simulink model "diff_flatness_linear_nl"  (R2022b)
settings: Solver=FixedStepAuto  StartTime=0.0  StopTime=15  RelTol=1e-3
model workspace (MAT data in the model file):
  kp = Simulink.Parameter
  kp.DataType = 'auto'
  kp.Complexity = 'real'
  kp.Dimensions = [0 0]
libraries: robotmobilelib x5, dspsigops x5
settings Model: Creator=RichiRettore  LastModifiedBy=RichiRettore
settings OptimizationCC: ReuseModelBlockBuffer=on

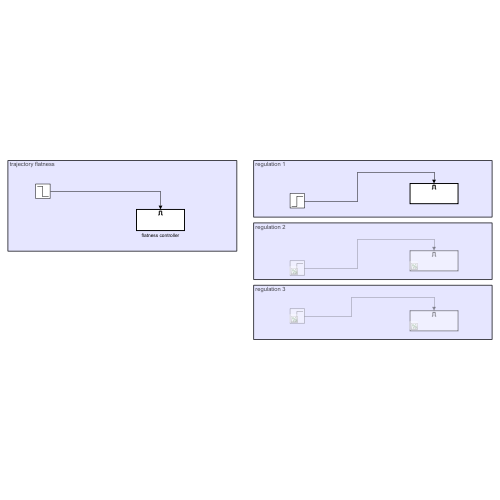
[thumbnail: Simulink's stored preview of the top-level diagram]
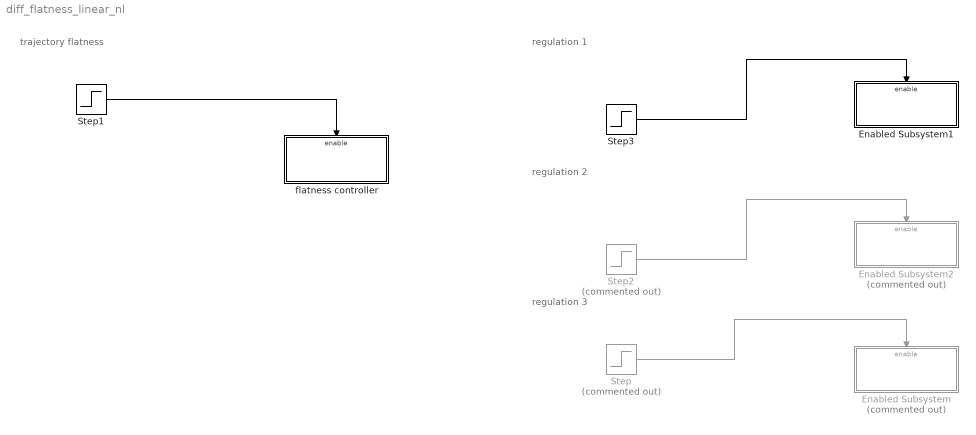
== system diff_flatness_linear_nl ==
  note: regulation 3
  note: regulation 2
  note: regulation 1
  note: trajectory flatness
  Enabled Subsystem : Subsystem  Commented=on  TreatAsAtomicUnit=on
  Enabled Subsystem1 : Subsystem  TreatAsAtomicUnit=on
  Enabled Subsystem2 : Subsystem  Commented=on  TreatAsAtomicUnit=on
  Step : Step  Commented=on  Time=10  SampleTime=0
  Step1 : Step  Time=10  Before=1  After=0  SampleTime=0
  Step2 : Step  Commented=on  Time=10  SampleTime=0
  Step3 : Step  Time=10  SampleTime=0
  flatness controller : Subsystem  TreatAsAtomicUnit=on
  wires:
  Step2/1 -> Enabled Subsystem2/Enable
  Step1/1 -> flatness controller/Enable
  Step/1 -> Enabled Subsystem/Enable
  Step3/1 -> Enabled Subsystem1/Enable

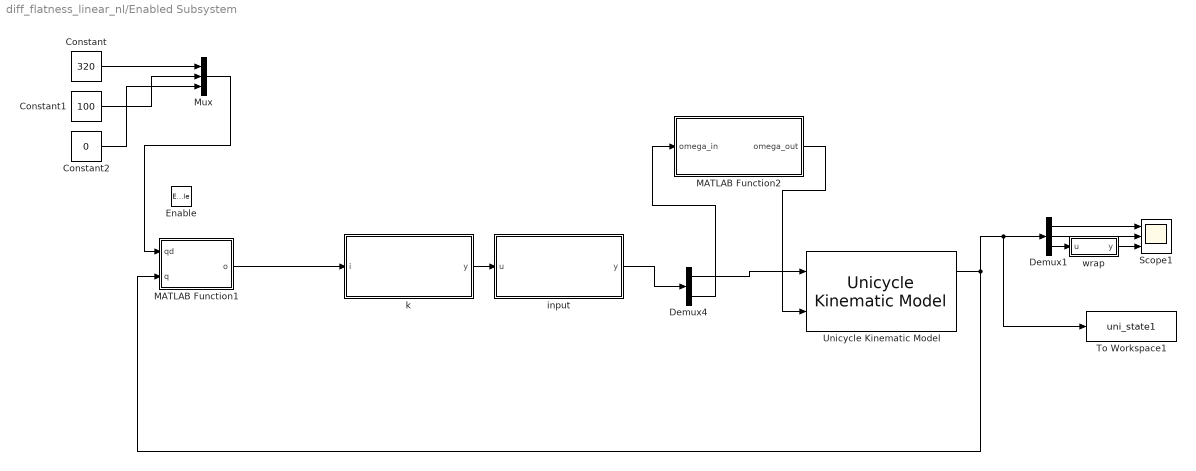
== system diff_flatness_linear_nl/Enabled Subsystem ==
  Enable : EnablePort
  Constant : Constant  Value=320
  Constant1 : Constant  Value=100
  Constant2 : Constant  Value=0
  Demux1 : Demux  Outputs=3
  Demux4 : Demux  Outputs=2
  MATLAB Function1 : MATLAB Function  TreatAsAtomicUnit=on
  MATLAB Function2 : MATLAB Function  TreatAsAtomicUnit=on
  Mux : Mux  Inputs=3
  Scope1 : Scope  NumInputPorts=3
  To Workspace1 : ToWorkspace  VariableName=uni_state1  SaveFormat=Structure With Time  SampleTime=0.001
  Unicycle Kinematic Model : robotmobilelib/Unicycle Kinematic Model  VehicleInputs=Vehicle Speed & Heading Angular Velocity  WheelRadius=2  WheelSpeedRange=[-Inf Inf]  InitialState=[125,60,0]  SimulateUsing=Interpreted execution
  input : MATLAB Function  TreatAsAtomicUnit=on
  k : MATLAB Function  TreatAsAtomicUnit=on
  wrap : MATLAB Function  TreatAsAtomicUnit=on
  wires:
  Constant/1 -> Mux/1
  Constant1/1 -> Mux/2
  Constant2/1 -> Mux/3
  Demux1/2 -> Scope1/2
  wrap/1(y) -> Scope1/3
  Unicycle Kinematic Model/1 -> To Workspace1/1, Demux1/1, MATLAB Function1/2(q)
  input/1(y) -> Demux4/1
  Demux1/3 -> wrap/1(u)
  k/1(y) -> input/1(u)
  Demux1/1 -> Scope1/1
  MATLAB Function1/1(o) -> k/1(i)
  Demux4/1 -> Unicycle Kinematic Model/1
  Mux/1 -> MATLAB Function1/1(qd)
  Demux4/2 -> MATLAB Function2/1(omega_in)
  MATLAB Function2/1(omega_out) -> Unicycle Kinematic Model/2

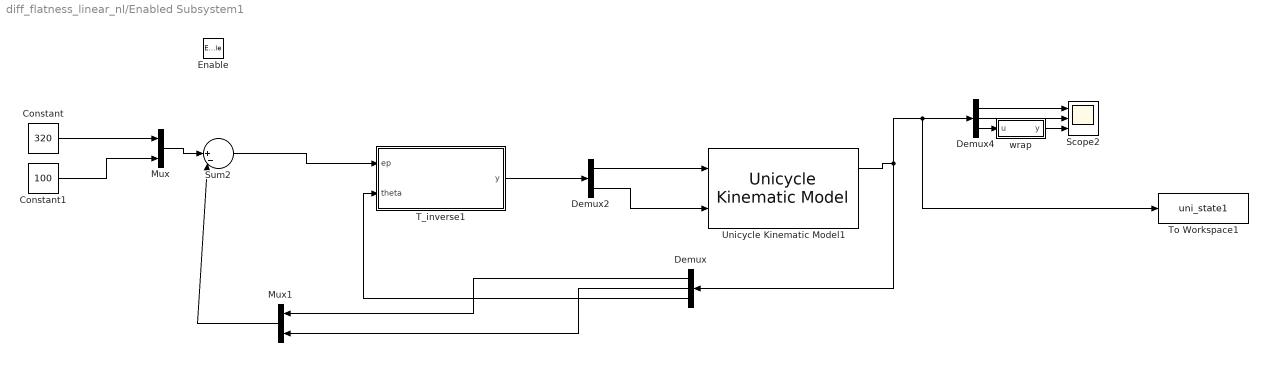
== system diff_flatness_linear_nl/Enabled Subsystem1 ==
  Enable : EnablePort
  Constant : Constant  Value=320
  Constant1 : Constant  Value=100
  Demux : Demux  Outputs=3
  Demux2 : Demux  Outputs=2
  Demux4 : Demux  Outputs=3
  Mux : Mux  Inputs=2
  Mux1 : Mux  Inputs=2
  Scope2 : Scope  NumInputPorts=3
  Sum2 : Sum  Inputs=||+-|
  T_inverse1 : MATLAB Function  TreatAsAtomicUnit=on
  To Workspace1 : ToWorkspace  VariableName=uni_state1  SaveFormat=Structure With Time  SampleTime=0.001
  Unicycle Kinematic Model1 : robotmobilelib/Unicycle Kinematic Model  VehicleInputs=Vehicle Speed & Heading Angular Velocity  WheelRadius=2  WheelSpeedRange=[-Inf Inf]  InitialState=[125,60,0]  SimulateUsing=Interpreted execution
  wrap : MATLAB Function  TreatAsAtomicUnit=on
  wires:
  wrap/1(y) -> Scope2/3
  Demux4/1 -> Scope2/1
  Demux4/2 -> Scope2/2
  Demux4/3 -> wrap/1(u)
  Sum2/1 -> T_inverse1/1(ep)
  Demux/1 -> Mux1/1
  Demux2/2 -> Unicycle Kinematic Model1/2
  Mux1/1 -> Sum2/2
  Demux2/1 -> Unicycle Kinematic Model1/1
  Unicycle Kinematic Model1/1 -> To Workspace1/1, Demux4/1, Demux/1
  T_inverse1/1(y) -> Demux2/1
  Demux/2 -> Mux1/2
  Demux/3 -> T_inverse1/2(theta)
  Constant1/1 -> Mux/2
  Constant/1 -> Mux/1
  Mux/1 -> Sum2/1

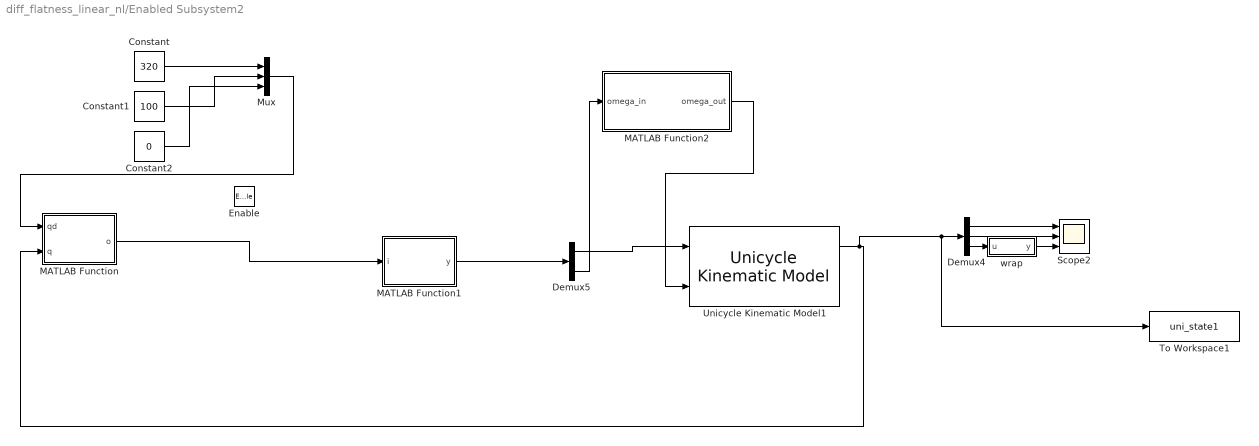
== system diff_flatness_linear_nl/Enabled Subsystem2 ==
  Enable : EnablePort
  Constant : Constant  Value=320
  Constant1 : Constant  Value=100
  Constant2 : Constant  Value=0
  Demux4 : Demux  Outputs=3
  Demux5 : Demux  Outputs=2
  MATLAB Function : MATLAB Function  TreatAsAtomicUnit=on
  MATLAB Function1 : MATLAB Function  TreatAsAtomicUnit=on
  MATLAB Function2 : MATLAB Function  TreatAsAtomicUnit=on
  Mux : Mux  Inputs=3
  Scope2 : Scope  NumInputPorts=3
  To Workspace1 : ToWorkspace  VariableName=uni_state1  SaveFormat=Structure With Time  SampleTime=0.001
  Unicycle Kinematic Model1 : robotmobilelib/Unicycle Kinematic Model  VehicleInputs=Vehicle Speed & Heading Angular Velocity  WheelRadius=2  WheelSpeedRange=[-Inf Inf]  InitialState=[125,60,0]  SimulateUsing=Interpreted execution
  wrap : MATLAB Function  TreatAsAtomicUnit=on
  wires:
  Demux5/1 -> Unicycle Kinematic Model1/1
  wrap/1(y) -> Scope2/3
  MATLAB Function/1(o) -> MATLAB Function1/1(i)
  MATLAB Function1/1(y) -> Demux5/1
  Demux4/1 -> Scope2/1
  Demux4/2 -> Scope2/2
  Demux4/3 -> wrap/1(u)
  Unicycle Kinematic Model1/1 -> To Workspace1/1, Demux4/1, MATLAB Function/2(q)
  Constant/1 -> Mux/1
  Constant1/1 -> Mux/2
  Constant2/1 -> Mux/3
  Mux/1 -> MATLAB Function/1(qd)
  Demux5/2 -> MATLAB Function2/1(omega_in)
  MATLAB Function2/1(omega_out) -> Unicycle Kinematic Model1/2

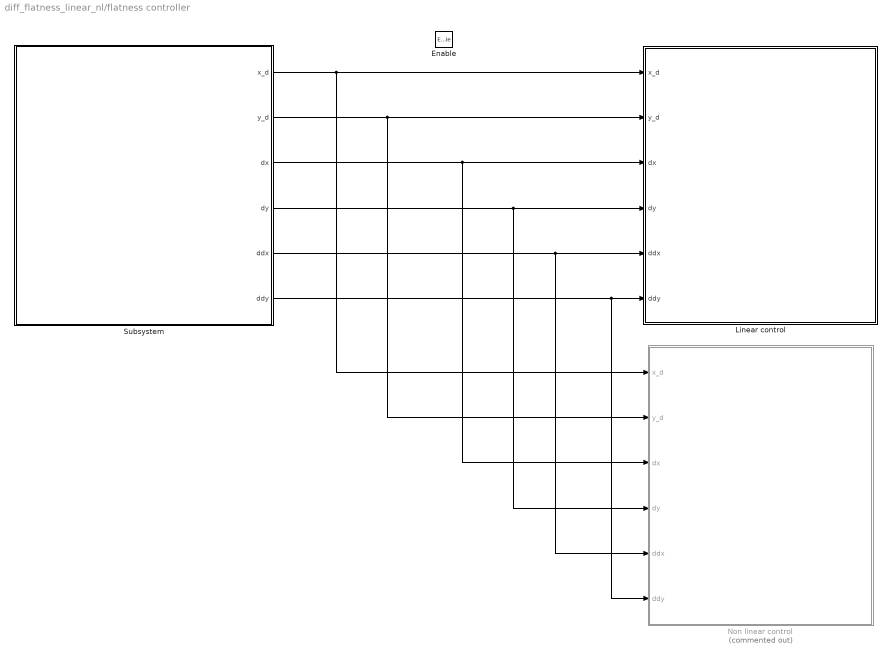
== system diff_flatness_linear_nl/flatness controller ==
  Enable : EnablePort
  Linear control : Subsystem
  Non linear control : Subsystem  Commented=on
  Subsystem : Subsystem
  wires:
  Subsystem/1(x_d) -> Non linear control/1(x_d), Linear control/1(x_d)
  Subsystem/2(y_d) -> Non linear control/2(y_d), Linear control/2(y_d)
  Subsystem/3(dx) -> Non linear control/3(dx), Linear control/3(dx)
  Subsystem/4(dy) -> Non linear control/4(dy), Linear control/4(dy)
  Subsystem/5(ddx) -> Non linear control/5(ddx), Linear control/5(ddx)
  Subsystem/6(ddy) -> Non linear control/6(ddy), Linear control/6(ddy)

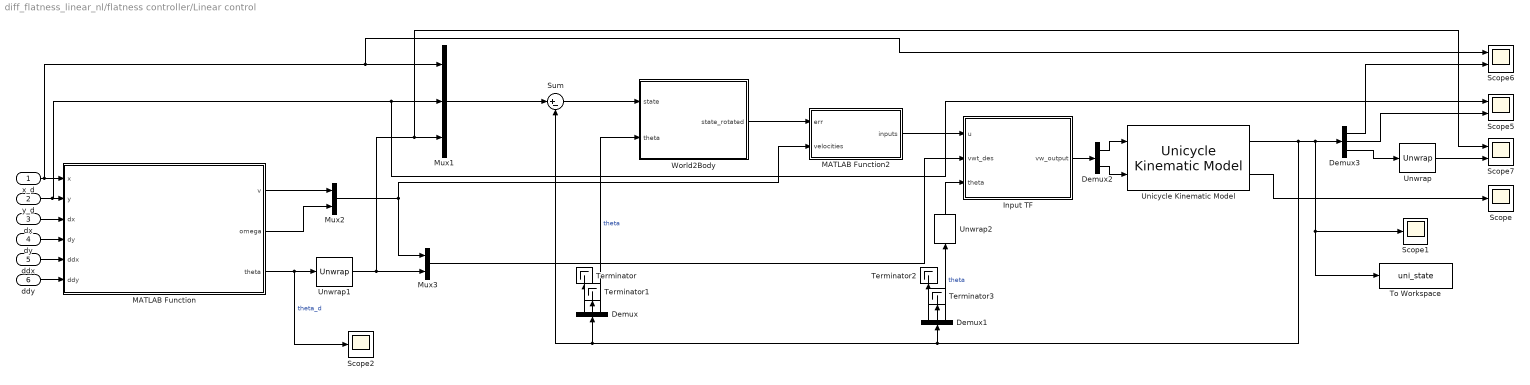
== system diff_flatness_linear_nl/flatness controller/Linear control ==
  x_d : Inport
  y_d : Inport  Port=2
  dx : Inport  Port=3
  dy : Inport  Port=4
  ddx : Inport  Port=5
  ddy : Inport  Port=6
  Demux : Demux  Outputs=3
  Demux1 : Demux  Outputs=3
  Demux2 : Demux  Outputs=2
  Demux3 : Demux  Outputs=3
  Input TF : MATLAB Function  TreatAsAtomicUnit=on
  MATLAB Function : MATLAB Function  TreatAsAtomicUnit=on
  MATLAB Function2 : MATLAB Function  TreatAsAtomicUnit=on
  Mux1 : Mux  Inputs=3
  Mux2 : Mux  Inputs=2
  Mux3 : Mux  Inputs=2
  Scope : Scope
  Scope1 : Scope
  Scope2 : Scope
  Scope5 : Scope  NumInputPorts=2
  Scope6 : Scope  NumInputPorts=2
  Scope7 : Scope  NumInputPorts=2
  Sum : Sum  Inputs=|+-
  Terminator{,1..3} (4 alike) : Terminator
  To Workspace : ToWorkspace  VariableName=uni_state  SaveFormat=Structure With Time  SampleTime=0.01
  Unicycle Kinematic Model : robotmobilelib/Unicycle Kinematic Model  VehicleInputs=Vehicle Speed & Heading Angular Velocity  WheelRadius=0.1  WheelSpeedRange=[-Inf Inf]  InitialState=[125; 60; 0]  SimulateUsing=Interpreted execution
  Unwrap : dspsigops/Unwrap  tol=pi  running=off
  Unwrap1 : dspsigops/Unwrap  tol=pi  running=off
  Unwrap2 : dspsigops/Unwrap  tol=pi  running=off
  World2Body : MATLAB Function  TreatAsAtomicUnit=on
  wires:
  Unicycle Kinematic Model/1 -> To Workspace/1, Scope1/1, Demux3/1, Sum/2, Demux/1, Demux1/1
  MATLAB Function/2(omega) -> Mux2/2
  dx/1 -> MATLAB Function/3(dx)
  Demux/3 -> World2Body/2(theta)  "theta"
  x_d/1 -> Scope6/1, Mux1/1, MATLAB Function/1(x)
  ddx/1 -> MATLAB Function/5(ddx)
  Sum/1 -> World2Body/1(state)
  World2Body/1(state_rotated) -> MATLAB Function2/1(err)
  Demux2/1 -> Unicycle Kinematic Model/1
  MATLAB Function2/1(inputs) -> Input TF/1(u)
  Demux2/2 -> Unicycle Kinematic Model/2
  Input TF/1(vw_output) -> Demux2/1
  Mux1/1 -> Sum/1
  MATLAB Function/3(theta) -> Unwrap1/1, Scope2/1  "theta_d"
  y_d/1 -> Scope5/1, Mux1/2, MATLAB Function/2(y)
  Demux3/1 -> Scope6/2
  Mux2/1 -> MATLAB Function2/2(velocities), Mux3/1
  Mux3/1 -> Input TF/2(vwt_des)
  Demux3/2 -> Scope5/2
  Unicycle Kinematic Model/2 -> Scope/1
  MATLAB Function/1(v) -> Mux2/1
  ddy/1 -> MATLAB Function/6(ddy)
  dy/1 -> MATLAB Function/4(dy)
  Demux/1 -> Terminator/1
  Demux/2 -> Terminator1/1
  Demux1/1 -> Terminator2/1
  Demux1/2 -> Terminator3/1
  Demux3/3 -> Unwrap/1
  Unwrap/1 -> Scope7/2
  Unwrap1/1 -> Scope7/1, Mux1/3, Mux3/2
  Demux1/3 -> Unwrap2/1  "theta"
  Unwrap2/1 -> Input TF/3(theta)

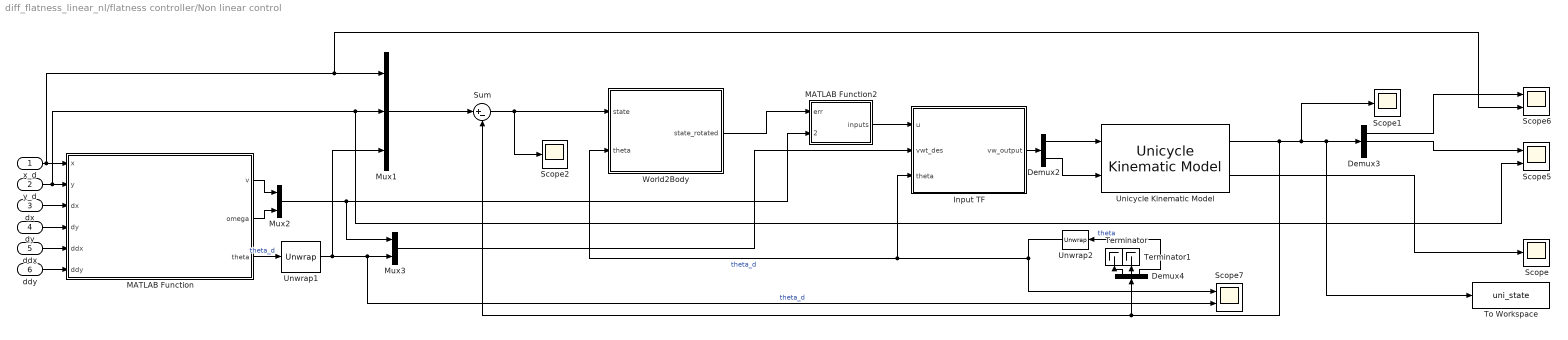
== system diff_flatness_linear_nl/flatness controller/Non linear control ==
  x_d : Inport
  y_d : Inport  Port=2
  dx : Inport  Port=3
  dy : Inport  Port=4
  ddx : Inport  Port=5
  ddy : Inport  Port=6
  Demux2 : Demux  Outputs=2
  Demux3 : Demux  Outputs=3
  Demux4 : Demux  Outputs=3
  Input TF : MATLAB Function  TreatAsAtomicUnit=on
  MATLAB Function : MATLAB Function  TreatAsAtomicUnit=on
  MATLAB Function2 : MATLAB Function  TreatAsAtomicUnit=on
  Mux1 : Mux  Inputs=3
  Mux2 : Mux  Inputs=2
  Mux3 : Mux  Inputs=2
  Scope : Scope
  Scope1 : Scope
  Scope2 : Scope
  Scope5 : Scope  NumInputPorts=2
  Scope6 : Scope  NumInputPorts=2
  Scope7 : Scope  NumInputPorts=2
  Sum : Sum  Inputs=|+-
  Terminator : Terminator
  Terminator1 : Terminator
  To Workspace : ToWorkspace  VariableName=uni_state  SaveFormat=Structure With Time  SampleTime=0.1
  Unicycle Kinematic Model : robotmobilelib/Unicycle Kinematic Model  VehicleInputs=Vehicle Speed & Heading Angular Velocity  WheelRadius=0.1  WheelSpeedRange=[-Inf Inf]  InitialState=[125; 60; 0]  SimulateUsing=Interpreted execution
  Unwrap1 : dspsigops/Unwrap  tol=pi  InputProcessing=Columns as channels (frame based)  running=off
  Unwrap2 : dspsigops/Unwrap  tol=pi  InputProcessing=Columns as channels (frame based)  running=off
  World2Body : MATLAB Function  TreatAsAtomicUnit=on
  wires:
  MATLAB Function/2(omega) -> Mux2/2
  dx/1 -> MATLAB Function/3(dx)
  x_d/1 -> Scope6/2, Mux1/1, MATLAB Function/1(x)
  ddx/1 -> MATLAB Function/5(ddx)
  Sum/1 -> World2Body/1(state), Scope2/1
  World2Body/1(state_rotated) -> MATLAB Function2/1(err)
  Demux2/1 -> Unicycle Kinematic Model/1
  MATLAB Function2/1(inputs) -> Input TF/1(u)
  Demux2/2 -> Unicycle Kinematic Model/2
  Input TF/1(vw_output) -> Demux2/1
  Mux1/1 -> Sum/1
  y_d/1 -> Scope5/2, Mux1/2, MATLAB Function/2(y)
  Demux3/1 -> Scope6/1
  Mux2/1 -> Mux3/1, MATLAB Function2/2(velocities)
  Mux3/1 -> Input TF/2(vwt_des)
  Demux3/2 -> Scope5/1
  Unicycle Kinematic Model/2 -> Scope/1
  MATLAB Function/1(v) -> Mux2/1
  ddy/1 -> MATLAB Function/6(ddy)
  dy/1 -> MATLAB Function/4(dy)
  MATLAB Function/3(theta) -> Unwrap1/1  "theta_d"
  Demux4/3 -> Unwrap2/1  "theta"
  Unwrap1/1 -> Mux1/3, Mux3/2, Scope7/2  "theta_d"
  Unicycle Kinematic Model/1 -> Demux4/1, Sum/2, To Workspace/1, Demux3/1, Scope1/1
  Unwrap2/1 -> Scope7/1, Input TF/3(theta), World2Body/2(theta)  "theta_d"
  Demux4/1 -> Terminator/1
  Demux4/2 -> Terminator1/1

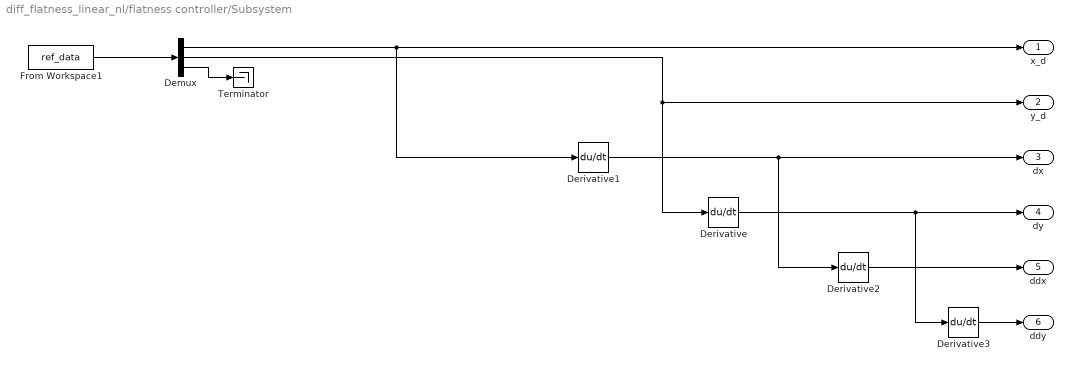
== system diff_flatness_linear_nl/flatness controller/Subsystem ==
  Demux : Demux  Outputs=3
  Derivative{,1..3} (4 alike) : Derivative
  From Workspace1 : FromWorkspace  VariableName=ref_data
  Terminator : Terminator
  x_d : Outport
  y_d : Outport  Port=2
  dx : Outport  Port=3
  dy : Outport  Port=4
  ddx : Outport  Port=5
  ddy : Outport  Port=6
  wires:
  Demux/3 -> Terminator/1
  Derivative/1 -> dy/1, Derivative3/1
  Derivative3/1 -> ddy/1
  Derivative1/1 -> dx/1, Derivative2/1
  From Workspace1/1 -> Demux/1
  Demux/1 -> x_d/1, Derivative1/1
  Demux/2 -> y_d/1, Derivative/1
  Derivative2/1 -> ddx/1

== matlab function diff_flatness_linear_nl/Enabled Subsystem/MATLAB Function2 ==
  data: omega_in input; omega_out output
function omega_out = check_omega(omega_in)
    % Check if omega (angular velocity) is finite
    if ~isfinite(omega_in)
        omega_out = 0;  % Set omega to a default value, e.g., 0 if it is NaN or Inf
    else
        omega_out = omega_in;  % Otherwise, pass the input value
    end
end

== matlab function diff_flatness_linear_nl/Enabled Subsystem/input ==
  data: u input; y output
function y = fcn(u)
v=u(2)*u(1);
w=u(3);
y = [v;w];

== matlab function diff_flatness_linear_nl/Enabled Subsystem/k ==
  data: i input; y output
function y = fcn(i)
k1=20;
k2=100;
k3=20;
rho=i(1);
gamma=i(2);
delta=i(3);
u=k1*cos(gamma);
w=k2*gamma+(k1* ((sin(gamma)*cos(gamma))/gamma) * (gamma+k3*delta));
y = [rho;u;w];

== matlab function diff_flatness_linear_nl/Enabled Subsystem/wrap ==
  data: u input; y output
function y = fcn(u)

y =mod(u+pi,2*pi)-pi;

== matlab function diff_flatness_linear_nl/Enabled Subsystem2/MATLAB Function ==
  data: qd input; o output; q input
function o = fcn(qd,q)
xi=q(1);
yi=q(2);
thetai=q(3);
x=-(qd(1)-xi);
y=-(qd(2)-yi);
theta=-(qd(3)-thetai);
rho=sqrt(x^2+y^2);
gamma=atan2(y,x)+pi-theta;
delta=gamma+theta;
delta=mod(delta+pi,2*pi)-pi;
gamma=mod(gamma+pi,2*pi)-pi;
o = [rho;gamma;delta];

== matlab function diff_flatness_linear_nl/Enabled Subsystem2/MATLAB Function1 ==
  data: i input; y output
function y = fcn(i)
k1=20;
k2=30;
k3=4;
rho=i(1);
gamma=i(2);
delta=i(3);
v=k1*rho*cos(gamma);
w=k2*gamma+(k1* ((sin(gamma)*cos(gamma))/gamma) * (gamma+k3*delta));
y = [v;w];

== matlab function diff_flatness_linear_nl/Enabled Subsystem1/wrap ==
  data: u input; y output
function y = fcn(u)

y =mod(u+pi,2*pi)-pi;

== matlab function diff_flatness_linear_nl/Enabled Subsystem1/T_inverse1 ==
  data: ep input; y output; theta input
function y = fcn(ep,theta)
theta=mod(theta+pi,2*pi)-pi;
kv=40;
kw=50;
v=kv*(ep(1)*cos(theta)+ep(2)*sin(theta));
w=kw*(atan2(-ep(2),-ep(1))+pi-theta);
y = [v;w];

== matlab function diff_flatness_linear_nl/flatness controller/Linear control/World2Body ==
  data: state input; state_rotated output; theta input
function state_rotated = rotation_matrix(state, theta)
% ROTATION_MATRIX Rotates the position [x; y] by an input angle theta.
%
% Inputs:
%   state - 3x1 vector representing [x; y; theta_state]
%   theta - Rotation angle in radians (scalar)
%
% Outputs:
%   state_rotated - 3x1 vector representing the rotated state [x_rot; y_rot; theta_state]

    % Extract x, y, and theta_state from the input state
    x = state(1);
    y = state(2);
    theta_state = state(3);

    % 2D rotation matrix for the x and y components
    R = [cos(theta), sin(theta);
         -sin(theta),  cos(theta)];

    % Rotate the [x; y] part of the state
    xy_rotated = R * [x; y];

    % Combine the rotated x, y, and the original theta_state into a 3x1 vector
    state_rotated = [xy_rotated; theta_state];
end

== matlab function diff_flatness_linear_nl/Enabled Subsystem2/MATLAB Function2 ==
  data: omega_in input; omega_out output
function omega_out = check_omega(omega_in)
    % Check if omega (angular velocity) is finite
    if ~isfinite(omega_in)
        omega_out = 0;  % Set omega to a default value, e.g., 0 if it is NaN or Inf
    else
        omega_out = omega_in;  % Otherwise, pass the input value
    end
end

== matlab function diff_flatness_linear_nl/Enabled Subsystem2/wrap ==
  data: u input; y output
function y = fcn(u)

y =mod(u+pi,2*pi)-pi;

== matlab function diff_flatness_linear_nl/flatness controller/Linear control/MATLAB Function ==
  data: x input; v output; omega output; y input; theta output; dx input; dy input; ddx input; ddy input
function [v, omega, theta] = unicycle_flatness_num(x, y, dx, dy, ddx, ddy)
    % Compute linear velocity safely
    velocity_magnitude = sqrt(dx^2 + dy^2);
    if velocity_magnitude < 1e-6
        v = 0;
    else
        v = velocity_magnitude;
    end

    % Compute heading angle
    theta = atan2(dy, dx);

    % Compute angular velocity safely
    denominator = dx^2 + dy^2;
    if denominator < 1e-6
        omega = 0;
    else
        omega = (dx * ddy - dy * ddx) / denominator;
    end
end

== matlab function diff_flatness_linear_nl/flatness controller/Linear control/Input TF ==
  data: u input; vwt_des input; vw_output output; theta input
function vw_output = input_transformation(u, vwt_des, theta)
% INPUT_TRANSFORMATION Computes the transformed velocities v and w.
%
% Inputs:
%   u        - 2x1 vector [u1; u2]
%   vwt_des  - 3x1 vector [v_des; w_des; theta_des]
%   theta    - Scalar rotation angle in radians
%
% Outputs:
%   vw_output - 2x1 vector [v; w] representing the transformed velocities

    % Extract inputs
    u1 = u(1);
    u2 = u(2);

    v_des = vwt_des(1);
    w_des = vwt_des(2);
    theta_des = vwt_des(3);

    % Compute the transformed velocities
    v = v_des * cos(theta_des - theta) - u1;
    w = w_des - u2;

    % Combine into a 2x1 output vector
    vw_output = [v; w];
end

== matlab function diff_flatness_linear_nl/flatness controller/Linear control/MATLAB Function2 ==
  data: err input; velocities input; inputs output
function inputs = fcn(err , velocities)
    d = 2 / sqrt(2);
    a = 15;
    vd = velocities(1);
    wd = velocities(2);
    
    % Safeguard for small vd
    vd_safe = sign(vd) * max(abs(vd), 1e-4);
    
    % Gains
    k1 = 2 * d * a;
    k2 = (a^2 - wd^2) / vd_safe;
    k3 = k1;
    
    % Clamp k2 to avoid large values
    max_k2 = 10;
    k2 = max(min(k2, max_k2), -max_k2);
    
    % Gain matrix
    k = [-k1, 0, 0;
         0, -k2, -k3];
    
    % Compute inputs and clamp to avoid excessively large values
    inputs = k * err;
    inputs = max(min(inputs, 10), -10);  % Clamping range for inputs
end

== matlab function diff_flatness_linear_nl/flatness controller/Non linear control/Input TF ==
  data: u input; vwt_des input; vw_output output; theta input
function vw_output = input_transformation(u, vwt_des, theta)
% INPUT_TRANSFORMATION Computes the transformed velocities v and w.
%
% Inputs:
%   u        - 2x1 vector [u1; u2]
%   vwt_des  - 3x1 vector [v_des; w_des; theta_des]
%   theta    - Scalar rotation angle in radians
%
% Outputs:
%   vw_output - 2x1 vector [v; w] representing the transformed velocities

    % Extract inputs
    u1 = u(1);
    u2 = u(2);

    v_des = vwt_des(1);
    w_des = vwt_des(2);
    theta_des = vwt_des(3);

    % Compute the transformed velocities
    v = v_des * cos(theta_des - theta) - u1;
    w = w_des - u2;

    % Combine into a 2x1 output vector
    vw_output = [v; w];
end

== matlab function diff_flatness_linear_nl/flatness controller/Non linear control/MATLAB Function ==
  data: x input; v output; omega output; y input; theta output; dx input; dy input; ddx input; ddy input
function [v, omega, theta] = unicycle_flatness_num(x, y, dx, dy, ddx, ddy)
    % Compute linear velocity safely
    velocity_magnitude = sqrt(dx^2 + dy^2);
    if velocity_magnitude < 1e-6
        v = 0;
    else
        v = velocity_magnitude;
    end

    % Compute heading angle
    theta = atan2(dy, dx);

    % Compute angular velocity safely
    denominator = dx^2 + dy^2;
    if denominator < 1e-6
        omega = 0;
    else
        omega = (dx * ddy - dy * ddx) / denominator;
    end
end

== matlab function diff_flatness_linear_nl/flatness controller/Non linear control/MATLAB Function2 ==
  data: err input; velocities input; inputs output
function inputs = fcn(err , velocities)
    d = 0.1 / sqrt(2);
    b = 0.5;
    vd = velocities(1);
    wd = velocities(2);
    e3 = err(3);

    % Safeguard for small vd
    e3 = sign(e3) * max(abs(e3), 1e-4);
    
    % Gains
    k1 = 2 * d * sqrt(b*vd+wd^2);
    k2 = b;
    k3 = k1;
    
    % Gain matrix
    k = [-k1, 0, 0;
         0, -k2*vd*(sin(e3)/e3), -k3];
    
    % Compute inputs and clamp to avoid excessively large values
    inputs = k * err;
    %inputs = max(min(inputs, 10), -10);  % Clamping range for inputs
end

== matlab function diff_flatness_linear_nl/flatness controller/Non linear control/World2Body ==
  data: state input; state_rotated output; theta input
function state_rotated = rotation_matrix(state, theta)
% ROTATION_MATRIX Rotates the position [x; y] by an input angle theta.
%
% Inputs:
%   state - 3x1 vector representing [x; y; theta_state]
%   theta - Rotation angle in radians (scalar)
%
% Outputs:
%   state_rotated - 3x1 vector representing the rotated state [x_rot; y_rot; theta_state]

    % Extract x, y, and theta_state from the input state
    x = state(1);
    y = state(2);
    theta_state = state(3);

    % 2D rotation matrix for the x and y components
    R = [cos(theta), sin(theta);
         -sin(theta),  cos(theta)];

    % Rotate the [x; y] part of the state
    xy_rotated = R * [x; y];

    % Combine the rotated x, y, and the original theta_state into a 3x1 vector
    state_rotated = [xy_rotated; theta_state];
end

== matlab function diff_flatness_linear_nl/Enabled Subsystem/MATLAB Function1 ==
  data: qd input; o output; q input
function o = fcn(qd,q)
xi=q(1);
yi=q(2);
thetai=q(3);
x=-(qd(1)-xi);
y=-(qd(2)-yi);
theta=-(qd(3)-thetai);
theta=mod(theta+pi,2*pi)-pi;
rho=sqrt(x^2+y^2);
gamma=atan2(y,x)+pi-theta;
delta=gamma+theta;
delta=mod(delta+pi,2*pi)-pi;
gamma=mod(gamma+pi,2*pi)-pi;
o = [rho;gamma;delta];
